simulink model "experimentA2"  (R2020a)
settings: Solver=FixedStepDiscrete  StartTime=0.0  StopTime=10.0  FixedStep=0.1  RelTol=1e-3  EnableMultiTasking=on
libraries: simulink x1
settings Model: Creator=hp-pc  LastModifiedBy=hp-pc
settings SolverCC: AutoInsertRateTranBlk=on
settings DataIOCC: LimitDataPoints=on
settings OptimizationCC: LifeSpan=inf
settings DebuggingCC: AllowSymbolicDim=off  SFUnexpectedBacktrackingDiag=warning  SFNoUnconditionalDefaultTransitionDiag=warning  SFExecutionAtInitializationDiag=none  ArithmeticOperatorsInVariantConditions=warning
settings SFSimCC: SimUseLocalCustomCode=off  CustomCodeUndefinedFunction=UseInterfaceOnly
settings RTWCC: RTWUseLocalCustomCode=off
settings CodeAppCC: StateflowObjectComments=on
settings GRTTargetCC: TargetLangStandard=C89/C90 (ANSI)
settings ConfigComp: CovMetricSettings=dw  CovHtmlReporting=on  CovSaveCumulativeToWorkspaceVar=on  CovSaveSingleToWorkspaceVar=on  CovShowResultsExplorer=off  CovExternalEMLEnable=off  CovSFcnEnable=off

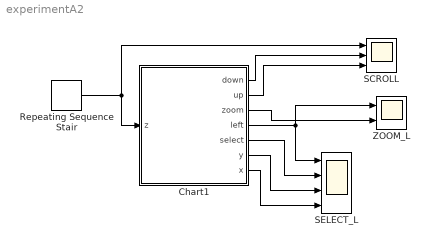
== system experimentA2 ==
  Chart1 : Stateflow chart  TreatAsAtomicUnit=on
      settings: PortSchema="{\"entries\":[{\"content\":{\"sides\":[{\"content\":{\"connectorIds\":[\"In1\"]},\"type\":\"ConnectorPlacement.EquallySpacedRectSide\",\"uuid\":\"b4c4336b-5a9f-49a8-ba4b-5e721e6ca1f7\"},{\"content\":{\"connectorIds\":[\"Out1\",\"Out2\",\"Out3\",\"Out7\",\"Out4\",\"Out5\",\"Out6\"],\"side\":\"RIGHT\"},\"type\":\"ConnectorPlacement.EquallySpacedRectSide\",\"uuid\":\"5d3eea68-70a9-4f4f-b9e8-d1fb1a9d7160\"},{\"content\":{\"connectorIds\":[],\"side\":\"TOP\"},\"type\":\"ConnectorPlacement.EquallySpacedRectSide\",\"uuid\":\"03f4b852-5b96-464b-bf16-c66fe05e7a4f\"}]},\"type\":\"ConnectorPlacement.EquallySpacedConnector\",\"uuid\":\"1a6a9704-51fc-42be-892e-bd1bb0d9d0c3\"}],\"packageUris\":[\"http://schema.mathworks.com/mf0/Connector/19700101\"],\"version\":\"1.0\"}"
  Repeating Sequence Stair : simulink/Sources/Repeating Sequence Stair  OutValues=[0 0 -1 1 0 1 0 0 -1 -1 1 0 1 0 -1].'  tsamp=-1  OutMin=[]  OutMax=[]  OutDataTypeStr=Inherit: Inherit via back propagation  OutDataType=fixdt(0,8)  ConRadixGroup=Best Precision: Vector-wise  OutScaling=2^-12
  SCROLL : Scope  NumInputPorts=3
  SELECT_L : Scope  NumInputPorts=4
  ZOOM_L : Scope  NumInputPorts=2
  wires:
  Chart1/6(x) -> SELECT_L/4
  Chart1/1(down) -> SCROLL/2
  Chart1/7(left) -> ZOOM_L/1, SELECT_L/1
  Repeating Sequence Stair/1 -> Chart1/1(z), SCROLL/1
  Chart1/5(y) -> SELECT_L/3
  Chart1/3(zoom) -> ZOOM_L/2
  Chart1/2(up) -> SCROLL/3
  Chart1/4(select) -> SELECT_L/2

== stateflow chart experimentA2/Chart1 ==
  state scroll_main
    state scroll
      down=0;
      up=0;
      z;
    state scroll_U
      entry:
      up=1;
    state scroll_D
      entry:
      down=1;
    (default) -> scroll
    scroll -> scroll_U [order 1] : [z==1]
    scroll_U -> scroll : after(2,sec){up=0;}
    scroll -> scroll_D [order 2] : [z==-1]
    scroll_D -> scroll : after(2,sec){down=0;}
  state Left_button_state
    state leftb1_select
      entry:
      select=1;
      x=1;
      y=1;
      left=1;
      l=1;
      du:l=l+1;
    state left_select1
      xi=1;yi=0;
      %both zero 4 zoom
      du:xi=xi+1;
      du:yi=yi+1;
      select=0;
      zoom=0;
    state left2_deselect
      entry:
      select=0;
      x=1;
      y=1;
      left=2;
    state leftb1_zoom_check
      entry:
      left=1;
      zoom=0;
      l=1;
      du:l=l+1;
    state leftb2_zoom_done
      entry:
      left=2;
      zoom=1;
    (default) -> left_select1
    left_select1 -> leftb1_select [order 1] : [((yi>0) || (xi>0))]%leftclick1_select
    leftb1_select -> left2_deselect : [(select==1)&&(l==2)]%left_deselect
    left2_deselect -> left_select1 : after(2,sec){left=0;}
    left_select1 -> leftb1_zoom_check [order 2] : [((yi==0) && (xi==0))]%double click zoom
    leftb1_zoom_check -> leftb2_zoom_done : before(2,sec)[l==2]%zoom_done
    leftb2_zoom_done -> left_select1 : after(2,sec){zoom=0;left=0}
  (default) -> scroll_main
  scroll -> Left_button_state [order 3] : [z==0]
  Left_button_state -> scroll : after(2,sec)[(z~=0)&&(left==0)]
  data: down output; up output; zoom output; select output; y output; x output; left output; xi local; yi local; z input; l local
